simulink model "chapter8_jd"  (R2016b)
settings: Solver=VariableStepAuto  StartTime=0.0  StopTime=10.0  RelTol=1e-3
settings Model: Creator=training-ah  LastModifiedBy=training-ah

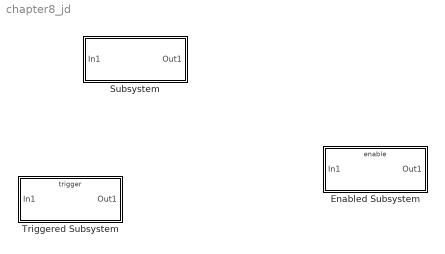
== system chapter8_jd ==
  Enabled Subsystem : Subsystem  TreatAsAtomicUnit=on
  Subsystem : Subsystem
  Triggered Subsystem : Subsystem  TreatAsAtomicUnit=on

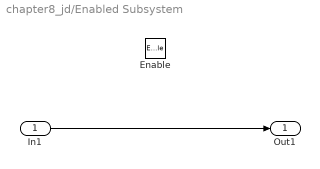
== system chapter8_jd/Enabled Subsystem ==
  In1 : Inport
  Enable : EnablePort
  Out1 : Outport
  wires:
  In1/1 -> Out1/1

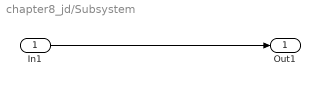
== system chapter8_jd/Subsystem ==
  In1 : Inport
  Out1 : Outport
  wires:
  In1/1 -> Out1/1

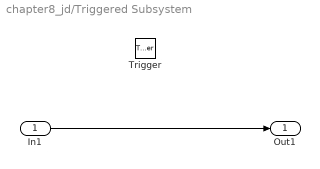
== system chapter8_jd/Triggered Subsystem ==
  In1 : Inport
  Trigger : TriggerPort  VariantControl=Variant
  Out1 : Outport
  wires:
  In1/1 -> Out1/1
